simulink model "EquationOfM"  (R2021b)
settings: Solver=VariableStepAuto  StartTime=0.0  StopTime=SimTime  RelTol=1e-3
values from neighbouring files (symbols this model uses):
  I = diag( [I_x I_y I_z ] )    [Lab_3.m]    (also in Lab_5.m)
  I_inv = inv( I )    [Lab_3.m]    (also in Lab_5.m)
  w_0 = [1e-6 1e-6 0.02]    [Lab_3.m]    (also in Lab_5.m = [ w_0x w_0y w_0z ])
libraries: vrlib x1
settings Model: Creator=adity  LastModifiedBy=adity
settings SolverCC: AlgebraicLoopSolver=TrustRegion
settings DebuggingCC: SFMachineParentedDataDiag=warning

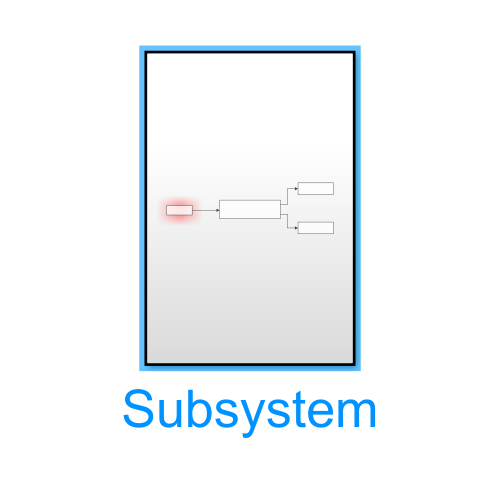
[thumbnail: Simulink's stored preview of the top-level diagram]
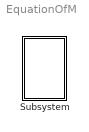
== system EquationOfM ==
  Subsystem : Subsystem

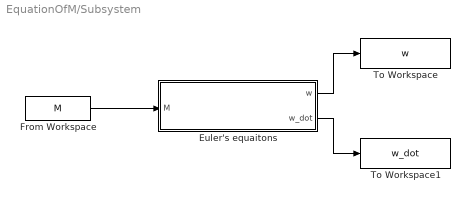
== system EquationOfM/Subsystem ==
  Euler's equaitons : Subsystem
  From Workspace : FromWorkspace  VariableName=M
  To Workspace : ToWorkspace  VariableName=w  SaveFormat=Timeseries  SampleTime=-1
  To Workspace1 : ToWorkspace  VariableName=w_dot  SaveFormat=Timeseries  SampleTime=-1
  wires:
  Euler's equaitons/2(w_dot) -> To Workspace1/1
  Euler's equaitons/1(w) -> To Workspace/1
  From Workspace/1 -> Euler's equaitons/1(M)

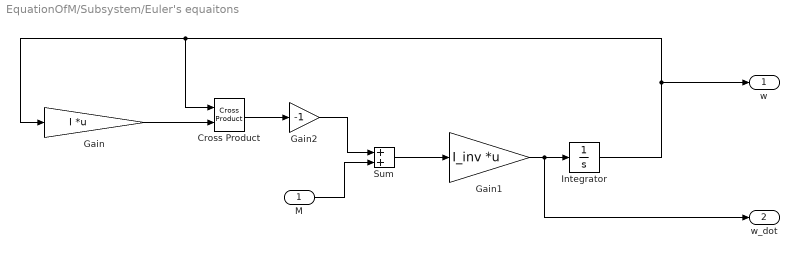
== system EquationOfM/Subsystem/Euler's equaitons ==
  M : Inport
  Cross Product : vrlib/Utilities/Cross Product
  Gain : Gain  Gain=I  Multiplication=Matrix(K*u) (u vector)
  Gain1 : Gain  Gain=I_inv  Multiplication=Matrix(K*u) (u vector)
  Gain2 : Gain  Gain=-1
  Integrator : Integrator  InitialCondition=w_0
  Sum : Sum
  w : Outport
  w_dot : Outport  Port=2
  wires:
  Gain2/1 -> Sum/1
  Cross Product/1 -> Gain2/1
  Gain1/1 -> w_dot/1, Integrator/1
  Integrator/1 -> w/1, Cross Product/1, Gain/1
  Gain/1 -> Cross Product/2
  Sum/1 -> Gain1/1
  M/1 -> Sum/2
